simulink model "Master"  (R2025b)
settings: Solver=VariableStepAuto  StartTime=0.0  StopTime=10.0  RelTol=1e-3
libraries: opcualib x1
settings Model: Creator=guilh  LastModifiedBy=guilh

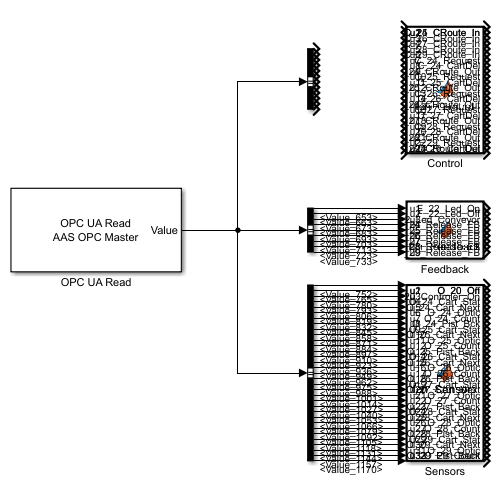
[thumbnail: Simulink's stored preview of the top-level diagram]
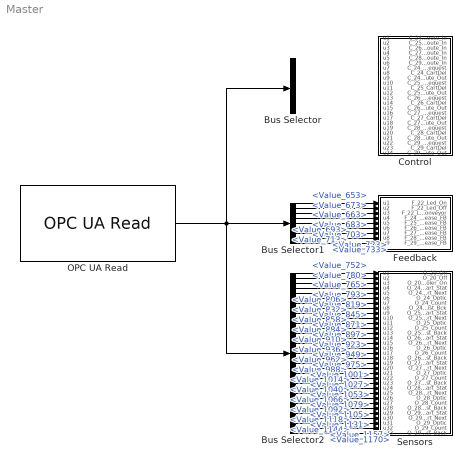
== system Master ==
  Bus Selector : BusSelector  OutputSignals=Value_527,Value_537,Value_547,Value_557,Value_567,Value_577,Value_587,Value_597,Value_607,Value_617,Value_627,Value_637
  Bus Selector1 : BusSelector  OutputSignals=Value_653,Value_663,Value_673,Value_683,Value_693,Value_703,Value_713,Value_723,Value_733
  Bus Selector2 : BusSelector  OutputSignals=Value_752,Value_765,Value_780,Value_793,Value_806,Value_819,Value_832,Value_845,Value_858,Value_871,Value_884,Value_897,Value_910,Value_923,Value_936,Value_949,Value_962,Value_975,Value_988,Value_1001,Value_1014,Value_1027,Value_1040,Value_1053,Value_1066,Value_1079,Value_1092,Value_1105,Value_1118,Value_1131,Value_1144,Value_1157,Value_1170
  Control : MATLAB Function  TreatAsAtomicUnit=on
  Feedback : MATLAB Function  TreatAsAtomicUnit=on
  OPC UA Read : opcualib/OPC UA Read  SelectedServer=AAS OPC Master  ServerList=AAS OPC Master  NodeList={ '1', 'Value', '6', '527', '1'; '2', 'Value', '6', '537', '1'; '3', 'Value', '6', '547', '1'; '4', 'Value', '6', '557', '1'; '5', 'Value', '6', '567', '1'; '6', 'Value', '6', '577', '1'; '7', 'Value', '6', '587', '1'; '8', 'Value', '6', '597', '1'; '9', 'Value', '6', '607', '1'; '10', 'Value', '6', '617', '1'; '11', 'Value', '6', '627', '1'; '12', 'Value', '6', '637', '1'; '13', 'Value', '6', '653', '1'; '14', 'Value', '6', '663', '1'; '15', 'Value', '6', '673', '1'; '16', 'Value', '6', '683', '1'; '17', 'Value', '6', '693', '1'; '18', 'Value', '6', '703', '1'; '19', 'Value', '6', '713', '1'; '20', 'Value', '6', '723', '1'; '21', 'Value', '6', '733', '1'; '22', 'Value', '6', '752', '1'; '23', 'Value', '6', '765', '1'; '24', 'Value', '6', '780', '1'; '25', 'Value', '6', '793', '1'; '26', 'Value', '6', '806', '1'; '27', 'Value', '6', '819', '1'; '28', 'Value', '6', '832', '1'; '29', 'Value', '6', '845', '1'; '30', 'Value', '6', '858', '1'; '31', 'Value', '6', '871', '1'; '32', 'Value', '6', '884', '1'; '33', 'Value', '6', '897', '1'; '34', 'Value', '6', '910', '1'; '35', 'Value', '6', '923', '1'; '36', 'Value', '6', '936', '1'; '37', 'Value', '6', '949', '1'; '38', 'Value', '6', '962', '1'; '39', 'Value', '6', '975', '1'; '40', 'Value', '6', '988', '1'; '41', 'Value', '6', '1001', '1'; '42', 'Value', '6', '1014', '1'; '43', 'Value', '6', '1027', '1'; '44', 'Value', '6', '1040', '1'; '45', 'Value', '6', '1053', '1'; '46', 'Value', '6', '1066', '1'; '47', 'Value', '6', '1079', '1'; '48', 'Value', '6', '1092', '1'; '49', 'Value', '6', '1105', '1'; '50', 'Value', '6', '1118', '1'; '51', 'Value', '6', '1131', '1'; '52', 'Value', '6', '1144', '1'; '53', 'Value', '6', '1157', '1'; '54', 'Value', '6', '1170', '1' }  ShowQualityPort=off  ShowTimestampPort=off  ShowTimestampPortAs=Seconds since start  SampleTime=-1
  Sensors : MATLAB Function  TreatAsAtomicUnit=on
  wires:
  OPC UA Read/1 -> Bus Selector2/1, Bus Selector1/1, Bus Selector/1
  Bus Selector1/1 -> Feedback/1(u1)  "<Value_653>"
  Bus Selector1/2 -> Feedback/2(u2)  "<Value_663>"
  Bus Selector1/3 -> Feedback/3(u3)  "<Value_673>"
  Bus Selector1/4 -> Feedback/4(u4)  "<Value_683>"
  Bus Selector1/5 -> Feedback/5(u5)  "<Value_693>"
  Bus Selector1/6 -> Feedback/6(u6)  "<Value_703>"
  Bus Selector1/7 -> Feedback/7(u7)  "<Value_713>"
  Bus Selector1/8 -> Feedback/8(u8)  "<Value_723>"
  Bus Selector1/9 -> Feedback/9(u9)  "<Value_733>"
  Bus Selector2/1 -> Sensors/1(u1)  "<Value_752>"
  Bus Selector2/2 -> Sensors/2(u2)  "<Value_765>"
  Bus Selector2/3 -> Sensors/3(u3)  "<Value_780>"
  Bus Selector2/4 -> Sensors/4(u4)  "<Value_793>"
  Bus Selector2/5 -> Sensors/5(u5)  "<Value_806>"
  Bus Selector2/6 -> Sensors/6(u6)  "<Value_819>"
  Bus Selector2/7 -> Sensors/7(u7)  "<Value_832>"
  Bus Selector2/8 -> Sensors/8(u8)  "<Value_845>"
  Bus Selector2/9 -> Sensors/9(u9)  "<Value_858>"
  Bus Selector2/10 -> Sensors/10(u10)  "<Value_871>"
  Bus Selector2/11 -> Sensors/11(u11)  "<Value_884>"
  Bus Selector2/12 -> Sensors/12(u12)  "<Value_897>"
  Bus Selector2/13 -> Sensors/13(u13)  "<Value_910>"
  Bus Selector2/14 -> Sensors/14(u14)  "<Value_923>"
  Bus Selector2/15 -> Sensors/15(u15)  "<Value_936>"
  Bus Selector2/16 -> Sensors/16(u16)  "<Value_949>"
  Bus Selector2/17 -> Sensors/17(u17)  "<Value_962>"
  Bus Selector2/18 -> Sensors/18(u18)  "<Value_975>"
  Bus Selector2/19 -> Sensors/19(u19)  "<Value_988>"
  Bus Selector2/20 -> Sensors/20(u20)  "<Value_1001>"
  Bus Selector2/21 -> Sensors/21(u21)  "<Value_1014>"
  Bus Selector2/22 -> Sensors/22(u22)  "<Value_1027>"
  Bus Selector2/23 -> Sensors/23(u23)  "<Value_1040>"
  Bus Selector2/24 -> Sensors/24(u24)  "<Value_1053>"
  Bus Selector2/25 -> Sensors/25(u25)  "<Value_1066>"
  Bus Selector2/26 -> Sensors/26(u26)  "<Value_1079>"
  Bus Selector2/27 -> Sensors/27(u27)  "<Value_1092>"
  Bus Selector2/28 -> Sensors/28(u28)  "<Value_1105>"
  Bus Selector2/29 -> Sensors/29(u29)  "<Value_1118>"
  Bus Selector2/30 -> Sensors/30(u30)  "<Value_1131>"
  Bus Selector2/31 -> Sensors/31(u31)  "<Value_1144>"
  Bus Selector2/32 -> Sensors/32(u32)  "<Value_1157>"
  Bus Selector2/33 -> Sensors/33(u33)  "<Value_1170>"

== matlab function Master/Feedback ==
  data: u1 input; F_22_Led_On output; u2 input; u3 input; u4 input; u5 input; u6 input; u7 input; u8 input; u9 input; F_22_Led_Off output; F_22_Led_Conveyor output; F_24_Release_FB output; F_25_Release_FB output; F_26_Release_FB output; F_27_Release_FB output; F_28_Release_FB output; F_29_Release_FB output
function [F_22_Led_On,F_22_Led_Off,F_22_Led_Conveyor,F_24_Release_FB,...
    F_25_Release_FB,F_26_Release_FB,F_27_Release_FB,F_28_Release_FB,...
    F_29_Release_FB] = fcn_Feedback(u1,u2,u3,u4,u5,u6,u7,u8,u9)

F_22_Led_On = u1;
F_22_Led_Off = u2;
F_22_Led_Conveyor = u3;
F_24_Release_FB = u4;
F_25_Release_FB = u5;
F_26_Release_FB = u6;
F_27_Release_FB = u7;
F_28_Release_FB = u8;
F_29_Release_FB = u9;

== matlab function Master/Sensors ==
  data: u1 input; O_20_On output; u2 input; u3 input; u4 input; u5 input; u6 input; u7 input; u8 input; u9 input; u10 input; u11 input; u12 input; u13 input; u14 input; u15 input; u16 input; u17 input; u18 input; u19 input; u20 input; u21 input; u22 input; u23 input; u24 input; u25 input; u26 input; u27 input; u28 input; u29 input; u30 input; u31 input; u32 input; u33 input; O_20_Off output; O_20_Controler_On output; O_24_Cart_Stat output; O_24_Cart_Next output; O_24_Optic output; O_24_Count output; O_24_Pist_Bck output; O_25_Cart_Stat output; O_25_Cart_Next output; O_25_Optic output; O_25_Count output; O_25_Pist_Back output; O_26_Cart_Stat output; O_26_Cart_Next output; O_26_Optic output; O_26_Count output; O_26_Pist_Back output; O_27_Cart_Stat output; O_27_Cart_Next output; O_27_Optic output; O_27_Count output; O_27_Pist_Back output; O_28_Cart_Stat output; O_28_Cart_Next output; O_28_Optic output; O_28_Count output; O_28_Pist_Back output; O_29_Cart_Stat output; O_29_Cart_Next output; O_29_Optic output; O_29_Count output; O_29_Pist_Back output
function [O_20_On,O_20_Off,O_20_Controler_On,...
    O_24_Cart_Stat,O_24_Cart_Next,O_24_Optic,O_24_Count,O_24_Pist_Bck,...
    O_25_Cart_Stat,O_25_Cart_Next,O_25_Optic,O_25_Count,O_25_Pist_Back,...
    O_26_Cart_Stat,O_26_Cart_Next,O_26_Optic,O_26_Count,O_26_Pist_Back,...
    O_27_Cart_Stat,O_27_Cart_Next,O_27_Optic,O_27_Count,O_27_Pist_Back,...
    O_28_Cart_Stat,O_28_Cart_Next,O_28_Optic,O_28_Count,O_28_Pist_Back,...
    O_29_Cart_Stat,O_29_Cart_Next,O_29_Optic,O_29_Count,O_29_Pist_Back...
    ] = fcn_Sensors(u1,u2,u3,u4,u5,u6,u7,u8,u9,u10,u11,u12,u13,u14,...
    u15,u16,u17,u18,u19,u20,u21,u22,u23,u24,u25,u26,u27,u28,u29,u30,...
    u31,u32,u33)

O_20_On            = u1;
O_20_Off           = u2;
O_20_Controler_On  = u3;

O_24_Cart_Stat     = u4;
O_24_Cart_Next     = u5;
O_24_Optic         = u6;
O_24_Count         = u7;
O_24_Pist_Bck      = u8;

O_25_Cart_Stat     = u9;
O_25_Cart_Next     = u10;
O_25_Optic         = u11;
O_25_Count         = u12;
O_25_Pist_Back     = u13;

O_26_Cart_Stat     = u14;
O_26_Cart_Next     = u15;
O_26_Optic         = u16;
O_26_Count         = u17;
O_26_Pist_Back     = u18;

O_27_Cart_Stat     = u19;
O_27_Cart_Next     = u20;
O_27_Optic         = u21;
O_27_Count         = u22;
O_27_Pist_Back     = u23;

O_28_Cart_Stat     = u24;
O_28_Cart_Next     = u25;
O_28_Optic         = u26;
O_28_Count         = u27;
O_28_Pist_Back     = u28;

O_29_Cart_Stat     = u29;
O_29_Cart_Next     = u30;
O_29_Optic         = u31;
O_29_Count         = u32;
O_29_Pist_Back     = u33;

== matlab function Master/Control ==
  data: u1 input; u2 input; u3 input; u4 input; u5 input; u6 input; u7 input; u8 input; u9 input; u10 input; u11 input; u12 input; C_24_CRoute_In output; C_25_CRoute_In output; C_26_CRoute_In output; C_27_CRoute_In output; C_28_CRoute_In output; C_29_CRoute_In output; C_24_Request output; C_24_CartDel output; C_24_CRoute_Out output; C_25_Request output; C_25_CartDel output; C_25_CRoute_Out output; C_26_Request output; C_26_CartDel output; C_26_CRoute_Out output; C_27_Request output; C_27_CartDel output; C_27_CRoute_Out output; C_28_Request output; C_28_CartDel output; C_28_CRoute_Out output; C_29_Request output; C_29_CartDel output; C_29_CRoute_Out output; u13 input; u14 input; u15 input; u16 input; u17 input; u18 input; u19 input; u20 input; u21 input; u22 input; u23 input; u24 input
function [C_24_CRoute_In,C_25_CRoute_In,C_26_CRoute_In,C_27_CRoute_In,...
C_28_CRoute_In,C_29_CRoute_In,C_24_Request,C_24_CartDel,C_24_CRoute_Out,...
C_25_Request,C_25_CartDel,C_25_CRoute_Out,C_26_Request,C_26_CartDel,...
C_26_CRoute_Out,C_27_Request,C_27_CartDel,C_27_CRoute_Out,C_28_Request,...
C_28_CartDel,C_28_CRoute_Out,C_29_Request,C_29_CartDel,C_29_CRoute_Out]...
= fcn_Control(u1,u2,u3,u4,u5,u6,u7,u8,u9,u10,u11,u12,u13,u14,u15,u16,...
u17,u18,u19,u20,u21,u22,u23,u24)

C_24_CRoute_In = u1;
C_25_CRoute_In = u2;
C_26_CRoute_In = u3;
C_27_CRoute_In = u4;
C_28_CRoute_In = u5;
C_29_CRoute_In = u6;
C_24_Request = u7;
C_24_CartDel = u8;
C_24_CRoute_Out = u9;
C_25_Request = u10;
C_25_CartDel = u11;
C_25_CRoute_Out = u12;
C_26_Request = u13;
C_26_CartDel = u14;
C_26_CRoute_Out = u15;
C_27_Request = u16;
C_27_CartDel = u17;
C_27_CRoute_Out = u18;
C_28_Request = u19;
C_28_CartDel = u20;
C_28_CRoute_Out = u21;
C_29_Request = u22;
C_29_CartDel = u23;
C_29_CRoute_Out = u24;
